simulink model "sampleModel1485_2_sub_sub"  (R2023a)
settings: Solver=VariableStepAuto  StartTime=0.0  StopTime=10.0  RelTol=1e-3
libraries: hdlsllib x4, simulink x2
settings Model: Creator=user1  LastModifiedBy=user1
settings OptimizationCC: BlockReduction=off  ConditionallyExecuteInputs=off

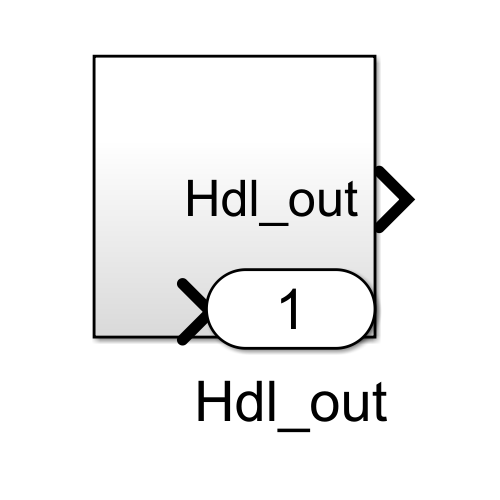
[thumbnail: Simulink's stored preview of the top-level diagram]
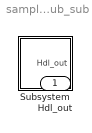
== system sampleModel1485_2_sub_sub ==
  Subsystem : Subsystem
  Hdl_out : Outport  OutDataTypeStr=uint8

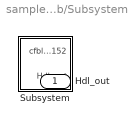
== system sampleModel1485_2_sub_sub/Subsystem ==
  Subsystem : Subsystem
  Hdl_out : Outport  OutDataTypeStr=uint8

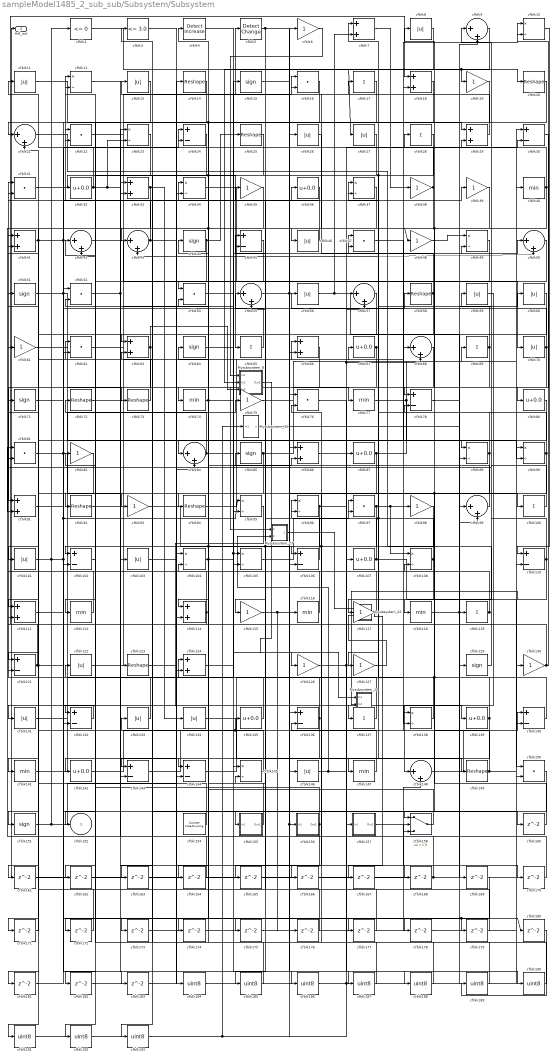
== system sampleModel1485_2_sub_sub/Subsystem/Subsystem ==
  Mysubsystem_10 : Subsystem  TreatAsAtomicUnit=on  RTWFcnName=Mysubsystem_10
      settings: RTWFcnNameOpts=User specified  RTWFileNameOpts=Use function name
  Mysubsystem_22 : Subsystem  TreatAsAtomicUnit=on  RTWFcnName=Mysubsystem_22
      settings: RTWFcnNameOpts=User specified  RTWFileNameOpts=Use function name
  Mysubsystem_27 : Subsystem  TreatAsAtomicUnit=on  RTWFcnName=Mysubsystem_27
      settings: RTWFcnNameOpts=User specified  RTWFileNameOpts=Use function name
  Mysubsystem_35 : Subsystem  TreatAsAtomicUnit=on  RTWFcnName=Mysubsystem_35
      settings: RTWFcnNameOpts=User specified  RTWFileNameOpts=Use function name
  Mysubsystem_8 : Subsystem  TreatAsAtomicUnit=on  RTWFcnName=Mysubsystem_8
      settings: RTWFcnNameOpts=User specified  RTWFileNameOpts=Use function name
  cfblk{10,12,23,34,37,49,89..90,95..96,104..105,108,138,145} (15 alike) : Product  Inputs=*/  OutDataTypeStr=uint8  RndMeth=Zero  SaturateOnIntegerOverflow=on
  cfblk{17,28,65,69,100,119,137} (7 alike) : Sum  Inputs=+  OutDataTypeStr=uint8
  cfblk{8,11,13,26..27,46,56,59..60,70,101,103,122,131,133..134,146} (17 alike) : Abs  OutDataTypeStr=uint8  SaturateOnIntegerOverflow=off
  cfblk{24,30,45,78,102,106,110,121,132,136,140,143..144} (13 alike) : Sum  Inputs=+-  OutDataTypeStr=uint8
  cfblk{32,36,67,80,87,107,135,139,142} (9 alike) : Bias  Bias=0.0  SaturateOnIntegerOverflow=off
  cfblk{7,18,29,33,41,63,66,86,91,111,114,124} (12 alike) : Sum  OutDataTypeStr=uint8
  cfblk{40,74,77,112,116,118,141,147} (8 alike) : MinMax  OutDataTypeStr=uint8
  cfblk{6,19,35,38..39,48,61,75,82,93,98,115,117,126..127,130} (16 alike) : Gain  OutDataTypeStr=uint8
  cfblk{14,20,25,58,72..73,92,94,123,149} (10 alike) : Reshape
  cfblk{15,44,51,64,71,85,129,151} (8 alike) : Signum
  cfblk{9,21,42..43,50,55,57,68,84,99,148} (11 alike) : Sum  Inputs=|++  OutDataTypeStr=uint8
  cfblk{16,22,31,47,52,54,62,76,81,97,150} (11 alike) : DotProduct  OutDataTypeStr=uint8
  cfblk154 : hdlsllib/Sources/Counter Free-Running  NumBits=16  tsamp=-1
  cfblk155 : Subsystem
      settings: LibrarySourceBlock=|
      | hdlsllib/Ports &
      | Subsystems/Subsystem
  cfblk156 : Subsystem
      settings: LibrarySourceBlock=|
      | hdlsllib/Ports &
      | Subsystems/Subsystem
  cfblk157 : Subsystem
      settings: LibrarySourceBlock=|
      | hdlsllib/Ports &
      | Subsystems/Subsystem
  cfblk158 : Switch  OutDataTypeStr=uint8  SaturateOnIntegerOverflow=off  InputSameDT=off
  cfblk{160..183} (24 alike) : Delay  SampleTime=1
  cfblk{184..193} (10 alike) : DataTypeConversion  OutDataTypeStr=uint8  SaturateOnIntegerOverflow=off  RndMeth=Floor
  cfblk2 : hdlsllib/Logic and Bit Operations/Compare To Zero  relop=<=  OutDataTypeStr=uint8
  cfblk3 : hdlsllib/Logic and Bit Operations/Compare To Constant  relop=<=  const=3.0  OutDataTypeStr=uint8
  cfblk4 : simulink/Logic and Bit Operations/Detect Increase  vinit=0.0  OutDataTypeStr=uint8
      settings: LibrarySourceBlock=|
      | hdlsllib/Logic and Bit
      | Operations/Detect
      | Increase
  cfblk5 : simulink/Logic and Bit Operations/Detect Change  vinit=0  OutDataTypeStr=uint8
      settings: LibrarySourceBlock=|
      | hdlsllib/Logic and Bit
      | Operations/Detect
      | Change
  cfblk152 : Outport  OutDataTypeStr=uint8  VectorParamsAs1DForOutWhenUnconnected=off
  Hdl_out : Outport  Port=2  OutDataTypeStr=uint8
  wires:
  Mysubsystem_35/1(y) -> cfblk119/1
  Mysubsystem_27/1(Out1) -> Mysubsystem_22/1(In1)
  Mysubsystem_22/1(Out1) -> cfblk167/1
  cfblk127/1 -> Mysubsystem_22/2(In2)
  Mysubsystem_8/1(Out1) -> Mysubsystem_10/1(In1)
  cfblk8/1 -> Mysubsystem_8/2(In2)
  cfblk6/1 -> Mysubsystem_8/1(In1)
  cfblk193/1 -> cfblk57/2
  cfblk150/1 -> cfblk193/1
  cfblk192/1 -> cfblk57/1
  cfblk169/1 -> cfblk192/1
  cfblk191/1 -> cfblk156/1(In1), cfblk6/1, Mysubsystem_35/1(In1)
  cfblk190/1 -> cfblk76/2
  cfblk189/1 -> cfblk76/1
  cfblk180/1 -> cfblk189/1
  cfblk188/1 -> cfblk82/1
  cfblk76/1 -> cfblk188/1
  cfblk187/1 -> cfblk4/1
  cfblk186/1 -> cfblk87/1, cfblk99/1
  cfblk185/1 -> cfblk3/1
  cfblk184/1 -> cfblk26/1
  cfblk3/1 -> cfblk184/1
  cfblk183/1 -> cfblk110/2
  cfblk182/1 -> cfblk84/2
  cfblk181/1 -> cfblk62/2
  cfblk179/1 -> cfblk41/2
  cfblk178/1 -> cfblk140/2
  cfblk177/1 -> cfblk12/2
  cfblk176/1 -> cfblk145/2
  cfblk175/1 -> cfblk158/3
  cfblk174/1 -> cfblk99/2
  cfblk173/1 -> cfblk150/2
  cfblk172/1 -> cfblk52/1
  cfblk24/1 -> cfblk172/1
  cfblk171/1 -> cfblk21/2
  cfblk170/1 -> cfblk136/1
  cfblk157/1(Out1) -> cfblk170/1
  cfblk168/1 -> cfblk33/1, Hdl_out/1
  cfblk92/1 -> cfblk168/1
  cfblk167/1 -> cfblk90/1
  cfblk166/1 -> cfblk96/2
  cfblk165/1 -> cfblk55/2
  cfblk164/1 -> cfblk81/1
  cfblk68/1 -> cfblk164/1
  cfblk163/1 -> cfblk158/2
  cfblk162/1 -> cfblk148/2
  cfblk161/1 -> cfblk104/1
  cfblk35/1 -> cfblk161/1
  cfblk160/1 -> cfblk86/1
  cfblk87/1 -> cfblk106/2, cfblk9/2
  cfblk104/1 -> cfblk86/2, cfblk54/2
  cfblk47/1 -> cfblk90/2
  cfblk131/1 -> cfblk15/1
  cfblk78/1 -> cfblk50/1
  cfblk90/1 -> cfblk106/1, cfblk37/2
  cfblk26/1 -> cfblk46/1
  cfblk140/1 -> cfblk8/1, cfblk47/1
  cfblk16/1 -> cfblk42/2
  cfblk11/1 -> cfblk33/2
  cfblk18/1 -> cfblk124/2
  cfblk4/1 -> cfblk186/1
  cfblk100/1 -> cfblk9/1
  cfblk142/1 -> cfblk30/1
  cfblk19/1 -> cfblk34/2, cfblk174/1
  cfblk143/1 -> cfblk18/2
  cfblk23/1 -> cfblk152/1
  cfblk75/1 -> cfblk77/1
  cfblk130/1 -> cfblk10/2, cfblk63/2
  cfblk111/1 -> cfblk58/1
  cfblk15/1 -> cfblk66/2
  cfblk41/1 -> cfblk37/1, cfblk160/1, cfblk151/1
  cfblk118/1 -> cfblk129/1, cfblk60/1
  cfblk49/1 -> cfblk73/1
  cfblk84/1 -> cfblk62/1, cfblk138/2
  cfblk25/1 -> cfblk94/1, cfblk43/1
  cfblk72/1 -> cfblk10/1
  cfblk158/1 -> cfblk64/1
  cfblk129/1 -> cfblk59/1
  cfblk126/1 -> cfblk68/2, cfblk50/2, cfblk157/1(In1)
  cfblk102/1 -> cfblk42/1
  cfblk124/1 -> cfblk16/1
  cfblk98/1 -> cfblk144/1, cfblk163/1, cfblk165/1
  cfblk50/1 -> cfblk63/1
  cfblk154/1 -> cfblk121/2
  cfblk101/1 -> cfblk95/1, cfblk24/2, cfblk178/1, cfblk2/1
  cfblk108/1 -> cfblk17/1, cfblk45/1, cfblk117/1
  cfblk42/1 -> cfblk116/1
  cfblk151/1 -> cfblk14/1, cfblk32/1
  cfblk38/1 -> cfblk74/1, cfblk28/1
  cfblk43/1 -> cfblk114/2, cfblk22/2
  cfblk134/1 -> cfblk149/1
  cfblk89/1 -> cfblk158/1, cfblk132/2, cfblk7/1
  cfblk61/1 -> cfblk123/1
  cfblk55/1 -> cfblk47/2, cfblk187/1
  cfblk80/1 -> cfblk101/1
  cfblk67/1 -> cfblk147/1, cfblk95/2
  cfblk115/1 -> cfblk176/1, cfblk177/1
  cfblk112/1 -> cfblk71/1
  cfblk71/1 -> cfblk155/1(In1)
  cfblk77/1 -> cfblk40/1, cfblk89/2
  cfblk103/1 -> cfblk67/1
  cfblk62/1 -> cfblk49/2
  cfblk10/1 -> cfblk110/1
  cfblk96/1 -> cfblk138/1, cfblk162/1
  cfblk32/1 -> cfblk23/2, cfblk144/2, cfblk11/1
  cfblk60/1 -> cfblk105/2
  cfblk56/1 -> cfblk7/2, cfblk169/1
  cfblk48/1 -> cfblk49/1
  cfblk13/1 -> cfblk21/1
  cfblk52/1 -> cfblk23/1, cfblk190/1
  cfblk110/1 -> Mysubsystem_10/2(In2), cfblk81/2
  cfblk136/1 -> cfblk85/1, cfblk182/1
  cfblk97/1 -> cfblk143/1, cfblk166/1, cfblk98/1, cfblk108/1
  cfblk58/1 -> cfblk121/1, cfblk16/2
  cfblk14/1 -> cfblk102/2
  cfblk30/1 -> cfblk80/1
  cfblk44/1 -> cfblk112/1, cfblk25/1
  cfblk135/1 -> cfblk72/1
  cfblk147/1 -> cfblk136/2
  cfblk107/1 -> cfblk150/1, cfblk45/2
  cfblk138/1 -> cfblk97/2
  cfblk36/1 -> cfblk31/2
  cfblk5/1 -> cfblk100/1, cfblk175/1
  cfblk93/1 -> cfblk146/1
  cfblk146/1 -> Mysubsystem_27/2(In2), cfblk30/2
  cfblk66/1 -> cfblk91/1
  cfblk86/1 -> cfblk107/1
  cfblk81/1 -> cfblk103/1, cfblk183/1
  cfblk133/1 -> cfblk122/1
  cfblk106/1 -> cfblk96/1
  cfblk117/1 -> cfblk61/1
  cfblk17/1 -> cfblk102/1
  cfblk137/1 -> cfblk124/1
  cfblk114/1 -> cfblk22/1, cfblk111/2
  cfblk139/1 -> cfblk142/1, cfblk108/2
  cfblk85/1 -> cfblk69/1, cfblk132/1
  cfblk9/1 -> cfblk27/1, cfblk19/1
  cfblk64/1 -> cfblk145/1
  cfblk91/1 -> cfblk34/1
  cfblk37/1 -> cfblk111/1, cfblk54/1
  cfblk45/1 -> cfblk93/1
  cfblk12/1 -> cfblk89/1
  cfblk69/1 -> cfblk114/1, cfblk43/2
  cfblk123/1 -> cfblk179/1, cfblk180/1
  cfblk70/1 -> Mysubsystem_27/1(In1), cfblk56/1
  cfblk116/1 -> cfblk35/1
  cfblk22/1 -> cfblk29/1
  cfblk149/1 -> cfblk130/1, cfblk78/2
  cfblk27/1 -> cfblk92/1
  cfblk40/1 -> cfblk12/1, cfblk143/2
  cfblk63/1 -> Mysubsystem_8/3(In3), cfblk171/1
  cfblk2/1 -> cfblk20/1
  cfblk122/1 -> cfblk5/1
  cfblk74/1 -> cfblk126/1, cfblk24/1
  cfblk34/1 -> cfblk70/1
  cfblk144/1 -> cfblk68/1
  cfblk155/1(Out1) -> cfblk104/2
  cfblk141/1 -> cfblk75/1
  cfblk99/1 -> cfblk52/2
  cfblk119/1 -> cfblk44/1, cfblk29/2
  cfblk54/1 -> cfblk105/1, cfblk137/1
  cfblk82/1 -> cfblk141/1
  cfblk73/1 -> cfblk41/1
  cfblk29/1 -> cfblk13/1
  cfblk65/1 -> cfblk55/1
  cfblk145/1 -> cfblk51/1, cfblk135/1
  cfblk95/1 -> cfblk133/1
  cfblk57/1 -> cfblk191/1
  cfblk39/1 -> cfblk48/1, cfblk78/1
  cfblk156/1(Out1) -> cfblk31/1, cfblk185/1
  cfblk94/1 -> cfblk66/1
  cfblk20/1 -> cfblk115/1
  cfblk46/1 -> cfblk36/1
  cfblk121/1 -> cfblk139/1, cfblk181/1, cfblk18/1
  cfblk51/1 -> cfblk84/1, cfblk39/1
  cfblk132/1 -> cfblk131/1
  cfblk28/1 -> cfblk127/1, cfblk173/1
  cfblk105/1 -> cfblk97/1
  cfblk59/1 -> cfblk148/1
  cfblk21/1 -> cfblk118/1
  cfblk148/1 -> cfblk140/1
  cfblk31/1 -> cfblk65/1
  cfblk7/1 -> cfblk38/1
  cfblk33/1 -> cfblk134/1, cfblk91/2

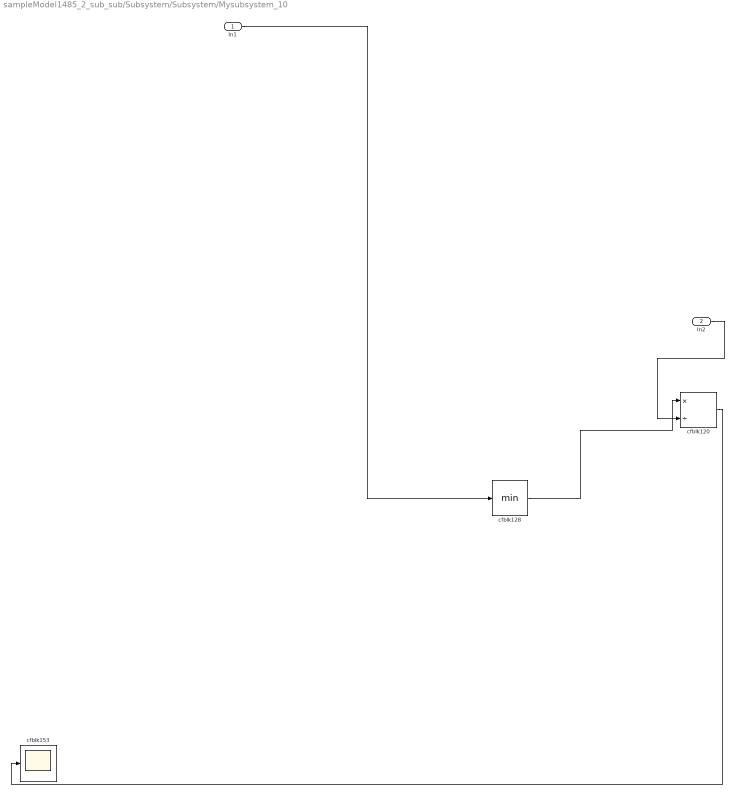
== system sampleModel1485_2_sub_sub/Subsystem/Subsystem/Mysubsystem_10 ==
  In1 : Inport
  In2 : Inport  Port=2
  cfblk120 : Product  Inputs=*/  RndMeth=Zero  SaturateOnIntegerOverflow=on
  cfblk128 : MinMax
  cfblk153 : Scope
  wires:
  cfblk128/1 -> cfblk120/1
  cfblk120/1 -> cfblk153/1
  In1/1 -> cfblk128/1
  In2/1 -> cfblk120/2

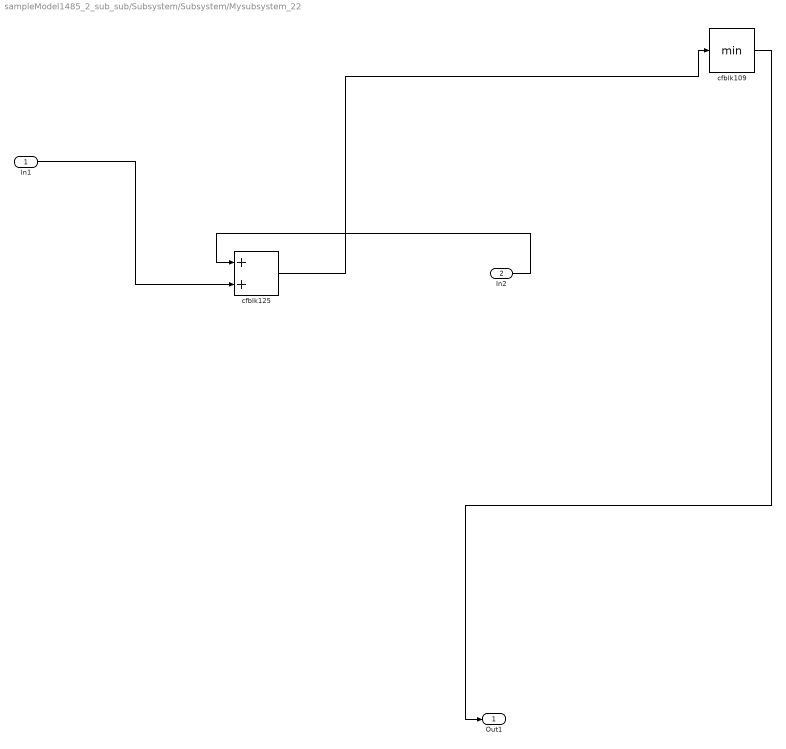
== system sampleModel1485_2_sub_sub/Subsystem/Subsystem/Mysubsystem_22 ==
  In1 : Inport
  In2 : Inport  Port=2
  cfblk109 : MinMax
  cfblk125 : Sum
  Out1 : Outport
  wires:
  cfblk125/1 -> cfblk109/1
  In1/1 -> cfblk125/2
  In2/1 -> cfblk125/1
  cfblk109/1 -> Out1/1

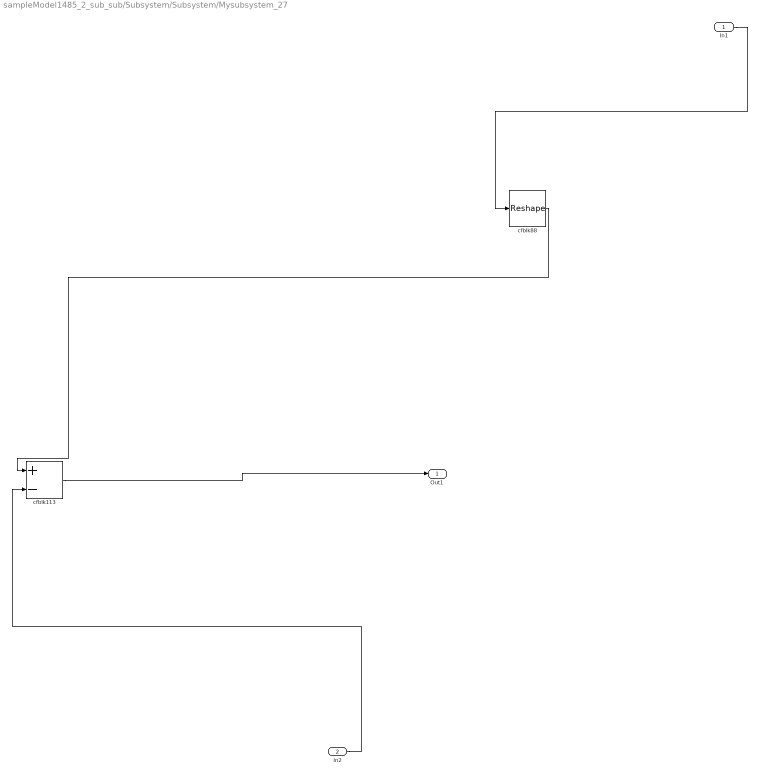
== system sampleModel1485_2_sub_sub/Subsystem/Subsystem/Mysubsystem_27 ==
  In1 : Inport
  In2 : Inport  Port=2
  cfblk113 : Sum  Inputs=+-
  cfblk88 : Reshape
  Out1 : Outport
  wires:
  cfblk88/1 -> cfblk113/1
  In1/1 -> cfblk88/1
  cfblk113/1 -> Out1/1
  In2/1 -> cfblk113/2

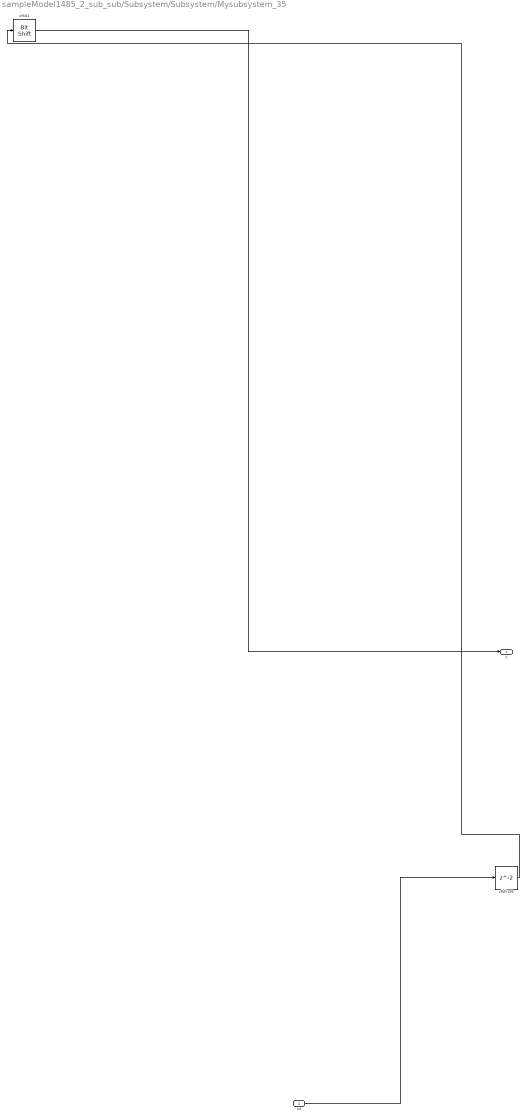
== system sampleModel1485_2_sub_sub/Subsystem/Subsystem/Mysubsystem_35 ==
  In1 : Inport
  cfblk1 : hdlsllib/Logic and Bit Operations/Bit Shift  mode=Shift Left Logical  N=0
  cfblk159 : Delay  SampleTime=1
  y : Outport
  wires:
  cfblk159/1 -> cfblk1/1
  cfblk1/1 -> y/1
  In1/1 -> cfblk159/1

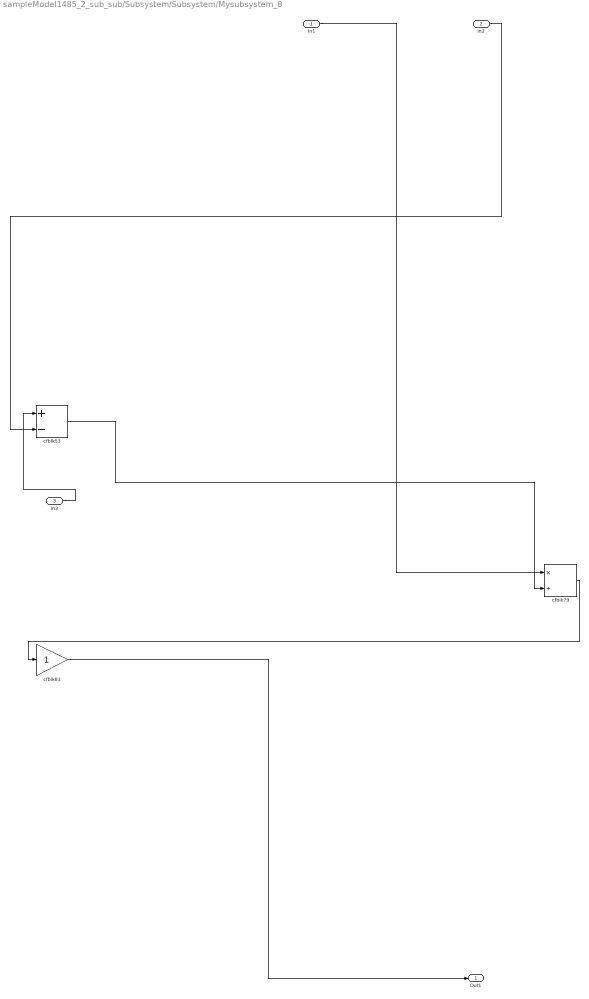
== system sampleModel1485_2_sub_sub/Subsystem/Subsystem/Mysubsystem_8 ==
  In1 : Inport
  In2 : Inport  Port=2
  In3 : Inport  Port=3
  cfblk53 : Sum  Inputs=+-
  cfblk79 : Product  Inputs=*/  RndMeth=Zero  SaturateOnIntegerOverflow=on
  cfblk83 : Gain
  Out1 : Outport
  wires:
  cfblk53/1 -> cfblk79/2
  cfblk83/1 -> Out1/1
  cfblk79/1 -> cfblk83/1
  In3/1 -> cfblk53/1
  In2/1 -> cfblk53/2
  In1/1 -> cfblk79/1

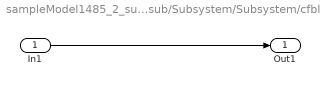
== system sampleModel1485_2_sub_sub/Subsystem/Subsystem/cfblk155 ==
  In1 : Inport
  Out1 : Outport
  wires:
  In1/1 -> Out1/1

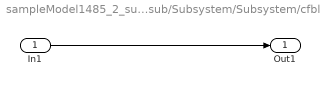
== system sampleModel1485_2_sub_sub/Subsystem/Subsystem/cfblk156 ==
  In1 : Inport
  Out1 : Outport
  wires:
  In1/1 -> Out1/1

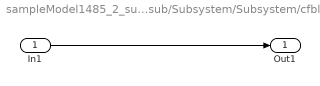
== system sampleModel1485_2_sub_sub/Subsystem/Subsystem/cfblk157 ==
  In1 : Inport
  Out1 : Outport
  wires:
  In1/1 -> Out1/1
